simulink model "Book6241"  (R2019b)
settings: Solver=ode4  StartTime=0.0  StopTime=50  FixedStep=0.001  RelTol=1e-3
settings Model: Creator=user  LastModifiedBy=user

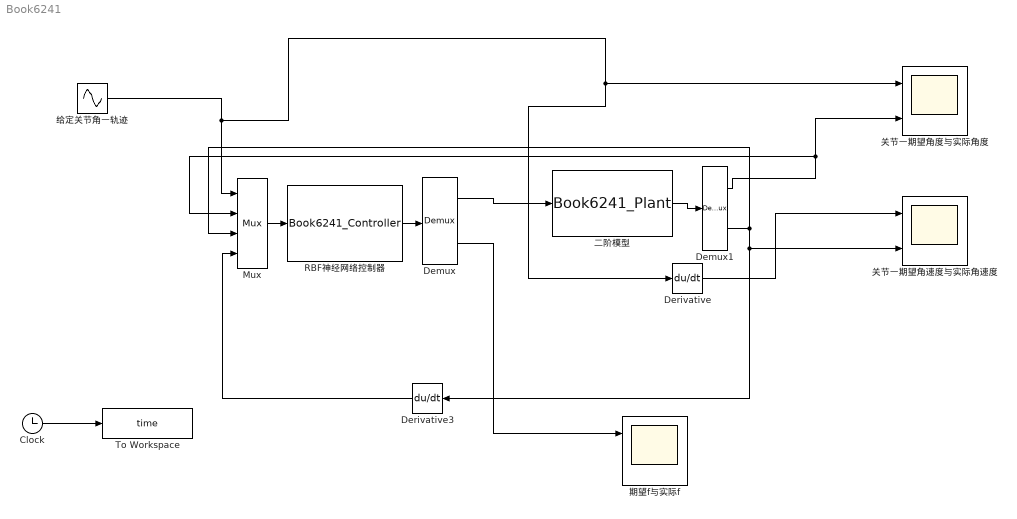
== system Book6241 ==
  Clock : Clock
  Demux : Demux  Outputs=2
  Demux1 : Demux  Outputs=2
  Derivative : Derivative
  Derivative3 : Derivative
  Mux : Mux
  RBF神经网络控制器 : S-Function  FunctionName=Book6241_Controller  SFunctionDeploymentMode=off  EnableBusSupport=off
  To Workspace : ToWorkspace  VariableName=time  SaveFormat=Timeseries  SampleTime=-1
  二阶模型 : S-Function  FunctionName=Book6241_Plant  SFunctionDeploymentMode=off  EnableBusSupport=off
  关节一期望角度与实际角度 : Scope  NumInputPorts=2
  关节一期望角速度与实际角速度 : Scope  NumInputPorts=2
  期望f与实际f : Scope  NumInputPorts=2
  给定关节角一轨迹 : Sin  SampleTime=0
  wires:
  Demux1/1 -> Mux/2, 关节一期望角度与实际角度/2
  Clock/1 -> To Workspace/1
  Demux/2 -> 期望f与实际f/1
  Derivative3/1 -> Mux/4
  RBF神经网络控制器/1 -> Demux/1
  Derivative/1 -> 关节一期望角速度与实际角速度/1
  Mux/1 -> RBF神经网络控制器/1
  Demux1/2 -> Mux/3, Derivative3/1, 关节一期望角速度与实际角速度/2
  给定关节角一轨迹/1 -> Derivative/1, 关节一期望角度与实际角度/1, Mux/1
  Demux/1 -> 二阶模型/1
  二阶模型/1 -> Demux1/1
